simulink model "test"  (R2018b)
settings: Solver=VariableStepAuto  StartTime=0.0  StopTime=10.0  RelTol=1e-3
values from neighbouring files (symbols this model uses):
  alpha = [-15 -14 -13 -12 -11 -10 -9 -8 -7 -6 -5 -4 ... (31 elements, 1x31)]    [flight_params.mat]
  cjet = [0 1 2 3 4 5 6 7 8 9 10 11 ... (21 elements, 1x21)]    [flight_params.mat]
  Cmtot = [0.4228 0.3198 0.2281 0.181 0.1563 0.1452 0.1431 0.1473 0.156 0.1681 0.1828 0.1996 ... (13671 elements, 21x21x31)]    [flight_params.mat]
  CXtot = [0.2676 0.6253 1.3667 2.1659 2.9949 3.8429 4.7045 5.5764 6.4565 7.3433 8.2357 9.1329 ... (13671 elements, 21x21x31)]    [flight_params.mat]
  CZtot = [1.463 1.7341 1.9204 2.0633 2.1859 2.2964 2.3987 2.4949 2.5867 2.6748 2.76 2.8429 ... (13671 elements, 21x21x31)]    [flight_params.mat]
  flap = [-10 -5 0 5 10 15 20 25 30 35 40 45 ... (21 elements, 1x21)]    [flight_params.mat]
settings Model: Creator=Alex  LastModifiedBy=Alex

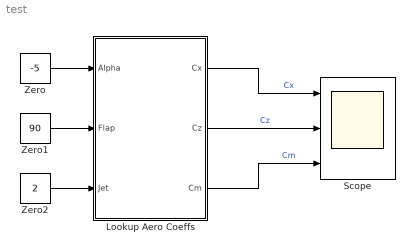
== system test ==
  Lookup Aero Coeffs : Subsystem
  Scope : Scope  NumInputPorts=3
  Zero : Constant  Value=-5  OutDataTypeStr=Inherit: Inherit via back propagation
  Zero1 : Constant  Value=90  OutDataTypeStr=Inherit: Inherit via back propagation
  Zero2 : Constant  Value=2  OutDataTypeStr=Inherit: Inherit via back propagation
  wires:
  Lookup Aero Coeffs/3(Cm) -> Scope/3  "Cm"
  Lookup Aero Coeffs/2(Cz) -> Scope/2  "Cz"
  Zero2/1 -> Lookup Aero Coeffs/3(Jet)
  Zero1/1 -> Lookup Aero Coeffs/2(Flap)
  Zero/1 -> Lookup Aero Coeffs/1(Alpha)
  Lookup Aero Coeffs/1(Cx) -> Scope/1  "Cx"

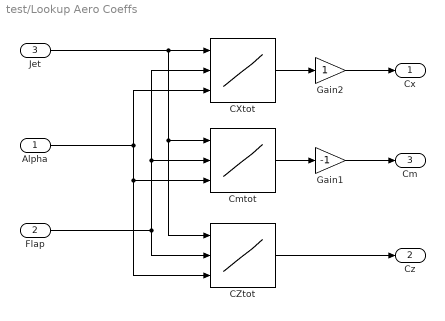
== system test/Lookup Aero Coeffs ==
  Alpha : Inport  Unit=rad
  Flap : Inport  Port=2  Unit=rad
  Jet : Inport  Port=3  Unit=rad
  CXtot : Lookup_n-D  NumberOfTableDimensions=3  BreakpointsForDimension1=cjet  BreakpointsForDimension2=flap  BreakpointsForDimension3=alpha  Table=CXtot  InternalRulePriority=Speed  RndMeth=Simplest  InputSameDT=on
  CZtot : Lookup_n-D  NumberOfTableDimensions=3  BreakpointsForDimension1=cjet  BreakpointsForDimension2=flap  BreakpointsForDimension3=alpha  Table=CZtot  InternalRulePriority=Speed  RndMeth=Simplest  InputSameDT=on
  Cmtot : Lookup_n-D  NumberOfTableDimensions=3  BreakpointsForDimension1=cjet  BreakpointsForDimension2=flap  BreakpointsForDimension3=alpha  Table=Cmtot  InternalRulePriority=Speed  RndMeth=Simplest  InputSameDT=on
  Gain1 : Gain  Gain=-1
  Gain2 : Gain
  Cx : Outport
  Cz : Outport  Port=2
  Cm : Outport  Port=3
  wires:
  Alpha/1 -> CXtot/3, CZtot/3, Cmtot/3
  Flap/1 -> CXtot/2, Cmtot/2, CZtot/2
  Jet/1 -> CZtot/1, Cmtot/1, CXtot/1
  CZtot/1 -> Cz/1
  Cmtot/1 -> Gain1/1
  Gain1/1 -> Cm/1
  CXtot/1 -> Gain2/1
  Gain2/1 -> Cx/1
